simulink model "model_xs_gen_data"  (R2022a)
settings: Solver=ode45  StartTime=6.69  StopTime=11.57  FixedStep=0.056  MaxStep=0.001  RelTol=1e-3  AbsTol=1e-3  EnableMultiTasking=on
values from neighbouring files (symbols this model uses):
  Fout = [0 0 0 0 0 0 0 0 0.0168265476136 0.0188041 0.0188041 0.00691430249089 ... (1118 elements, 1118x1)]    [generated_data.mat]
  k = par(:, 2)    [ga_error.m]    (also in ga_error_gen_data.m; ga_optim.m = ParOpt(2); ga_optim_gen_data.m = ParOpt(2); ga_rv_optim.m = ParOpt(2))
  k1 = par(:, 3)    [ga_error.m]    (also in ga_error_gen_data.m; ga_optim.m = ParOpt(3); ga_optim_gen_data.m = ParOpt(3); ga_rv_optim.m = ParOpt(3))
  mu = par(:, 1)    [ga_error.m]    (also in ga_error_gen_data.m; ga_optim.m = ParOpt(1); ga_optim_gen_data.m = ParOpt(1); ga_rv_optim.m = ParOpt(1))
  S0 = Sd(1)    [Input_data.m]    (also in Input_data_sim.m; ga_optim.m; ga_optim_gen_data.m; ga_rv_optim.m)
  So = 100    [Input_data.m]    (also in Input_data_sim.m; ga_optim.m; ga_optim_gen_data.m; ga_rv_optim.m)
  tfe = tfeed    [ga_optim_gen_data.m]    (also in ga_rv_optim_gen_data.m)
  Vout = [1.35 1.35 1.35 1.35 1.35 1.35 1.35 1.35 1.35003365292 1.3500702132 1.35010340908 1.350112825 ... (1118 elements, 1118x1)]    [generated_data.mat]
  X0 = Xd(1)    [Input_data.m]    (also in Input_data_sim.m; ga_optim.m; ga_optim_gen_data.m; ga_rv_optim.m)
settings Model: ExtModeTrigMode=oneshot  ExtModeArmWhenConnect=off  Creator=Olympia  LastModifiedBy=Olympia
settings SolverCC: AutoScaleAbsTol=off  AlgebraicLoopSolver=TrustRegion
settings DataIOCC: SaveFormat=Array  SignalLoggingSaveFormat=ModelDataLogs  SaveOutput=off  SaveTime=off  ReturnWorkspaceOutputs=off
settings OptimizationCC: BlockReduction=off  BooleanDataType=off
settings DebuggingCC: SaveWithParameterizedLinksMsg=none  UnderspecifiedInitializationDetection=Classic  MergeDetectMultiDrivingBlocksExec=none  SignalResolutionControl=TryResolveAllWithWarning  MultiTaskDSMMsg=warning  MultiTaskCondExecSysMsg=none  UnconnectedInputMsg=warning  UnconnectedOutputMsg=warning  UnconnectedLineMsg=warning  SFMachineParentedDataDiag=warning  ArithmeticOperatorsInVariantConditions=warning
settings HardwareCC: TargetUnknown=on
settings ModelReferenceCC: PropagateSignalLabelsOutOfModel=off
settings SFSimCC: SimUseLocalCustomCode=off  CustomCodeUndefinedFunction=UseInterfaceOnly
settings RTWCC: RTWUseLocalCustomCode=off
settings CodeAppCC: StateflowObjectComments=on
settings GRTTargetCC: TargetLangStandard=C89/C90 (ANSI)  CombineOutputUpdateFcns=off  GRTInterface=on

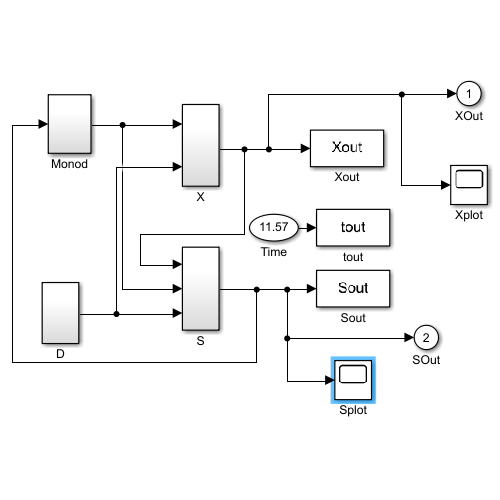
[thumbnail: Simulink's stored preview of the top-level diagram]
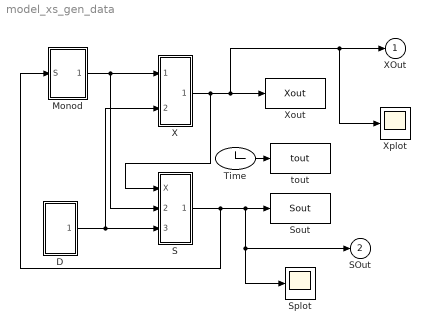
== system model_xs_gen_data ==
  D : Subsystem
  Monod : Subsystem
  S : Subsystem
  Sout : ToWorkspace  VariableName=Sout  SampleTime=-1
  Splot : Scope
  Time : Clock
  X : Subsystem
  Xout : ToWorkspace  VariableName=Xout  SampleTime=-1
  Xplot : Scope
  tout : ToWorkspace  VariableName=tout  SampleTime=-1
  XOut : Outport
  SOut : Outport  Port=2
  wires:
  X/1(XOut) -> Xout/1, Xplot/1, XOut/1, S/1(X)
  S/1(Sout) -> Monod/1(S), Sout/1, Splot/1, SOut/1
  Time/1 -> tout/1
  Monod/1(mu) -> X/1(mu), S/2(mu)
  D/1(out_1) -> S/3(F/V), X/2(F/V)

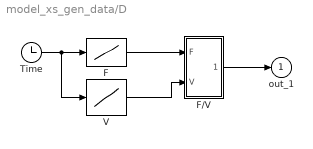
== system model_xs_gen_data/D ==
  F : Lookup  InputValues=tfe  Table=Fout
  F/V : Subsystem  mask(/){}
      mask help: Division of two scalars. y=u[1]/u[2]
      mask Help: Division of two scalars: y=u[1]/u[2]
      mask Display: disp('/')
  Time : Clock
  V : Lookup  InputValues=tfe  Table=Vout
  out_1 : Outport
  wires:
  F/V/1(out_1) -> out_1/1
  F/1 -> F/V/1(F)
  V/1 -> F/V/2(V)
  Time/1 -> F/1, V/1

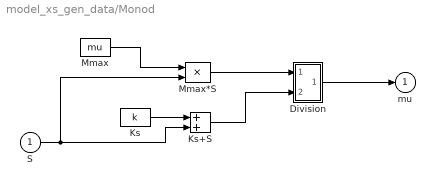
== system model_xs_gen_data/Monod ==
  S : Inport
  Division : Subsystem  mask(/){}
      mask help: Division of two scalars. y=u[1]/u[2]
      mask Help: Division of two scalars: y=u[1]/u[2]
      mask Display: disp('/')
  Ks : Constant  Value=k
  Ks+S : Sum  InputSameDT=on  SaturateOnIntegerOverflow=on  OutDataTypeStr=Inherit: Same as first input
  Mmax : Constant  Value=mu
  Mmax*S : Product  InputSameDT=on  RndMeth=Zero  SaturateOnIntegerOverflow=on  OutDataTypeStr=Inherit: Same as first input
  mu : Outport
  wires:
  Division/1(out_1) -> mu/1
  Mmax/1 -> Mmax*S/1
  Mmax*S/1 -> Division/1(Mmax*S)
  Ks+S/1 -> Division/2(Ks+S)
  Ks/1 -> Ks+S/1
  S/1 -> Ks+S/2, Mmax*S/2

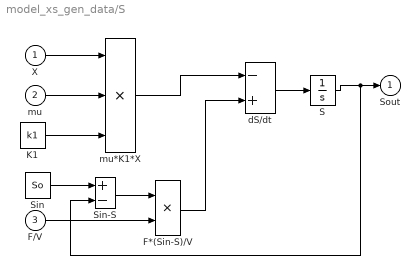
== system model_xs_gen_data/S ==
  X : Inport
  mu : Inport  Port=2
  F/V : Inport  Port=3
  F*(Sin-S)/V : Product  InputSameDT=on  RndMeth=Zero  SaturateOnIntegerOverflow=on  OutDataTypeStr=Inherit: Same as first input
  K1 : Constant  Value=k1
  S : Integrator  InitialCondition=S0  UpperSaturationLimit=1000  LowerSaturationLimit=0
  Sin : Constant  Value=So
  Sin-S : Sum  Inputs=+-  InputSameDT=on  SaturateOnIntegerOverflow=on  OutDataTypeStr=Inherit: Same as first input
  dS/dt : Sum  Inputs=-+  InputSameDT=on  SaturateOnIntegerOverflow=on  OutDataTypeStr=Inherit: Same as first input
  mu*K1*X : Product  Inputs=3  InputSameDT=on  RndMeth=Zero  SaturateOnIntegerOverflow=on  OutDataTypeStr=Inherit: Same as first input
  Sout : Outport
  wires:
  S/1 -> Sout/1, Sin-S/2
  Sin-S/1 -> F*(Sin-S)/V/1
  Sin/1 -> Sin-S/1
  X/1 -> mu*K1*X/1
  F/V/1 -> F*(Sin-S)/V/2
  mu*K1*X/1 -> dS/dt/1
  F*(Sin-S)/V/1 -> dS/dt/2
  dS/dt/1 -> S/1
  mu/1 -> mu*K1*X/2
  K1/1 -> mu*K1*X/3

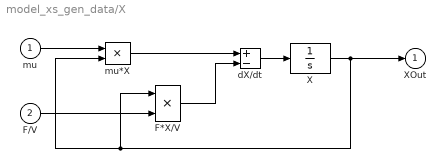
== system model_xs_gen_data/X ==
  mu : Inport
  F/V : Inport  Port=2
  F*X/V : Product  InputSameDT=on  RndMeth=Zero  SaturateOnIntegerOverflow=on  OutDataTypeStr=Inherit: Same as first input
  X : Integrator  InitialCondition=X0  UpperSaturationLimit=1000  LowerSaturationLimit=0
  dX/dt : Sum  Inputs=+-  InputSameDT=on  SaturateOnIntegerOverflow=on  OutDataTypeStr=Inherit: Same as first input
  mu*X : Product  InputSameDT=on  RndMeth=Zero  SaturateOnIntegerOverflow=on  OutDataTypeStr=Inherit: Same as first input
  XOut : Outport
  wires:
  F*X/V/1 -> dX/dt/2
  dX/dt/1 -> X/1
  mu*X/1 -> dX/dt/1
  mu/1 -> mu*X/1
  X/1 -> XOut/1, mu*X/2, F*X/V/1
  F/V/1 -> F*X/V/2

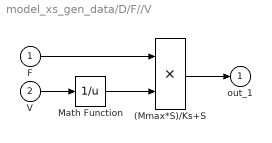
== system model_xs_gen_data/D/F//V ==
  F : Inport
  V : Inport  Port=2
  (Mmax*S)/Ks+S : Product  InputSameDT=on  RndMeth=Zero  SaturateOnIntegerOverflow=on  OutDataTypeStr=Inherit: Same as first input
  Math Function : Math  Operator=reciprocal  SignedPower=on
  out_1 : Outport
  wires:
  F/1 -> (Mmax*S)/Ks+S/1
  V/1 -> Math Function/1
  Math Function/1 -> (Mmax*S)/Ks+S/2
  (Mmax*S)/Ks+S/1 -> out_1/1

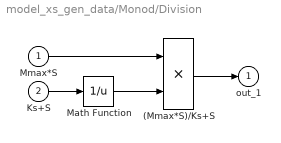
== system model_xs_gen_data/Monod/Division ==
  Mmax*S : Inport
  Ks+S : Inport  Port=2
  (Mmax*S)/Ks+S : Product  InputSameDT=on  RndMeth=Zero  SaturateOnIntegerOverflow=on  OutDataTypeStr=Inherit: Same as first input
  Math Function : Math  Operator=reciprocal  SignedPower=on
  out_1 : Outport
  wires:
  Mmax*S/1 -> (Mmax*S)/Ks+S/1
  Ks+S/1 -> Math Function/1
  Math Function/1 -> (Mmax*S)/Ks+S/2
  (Mmax*S)/Ks+S/1 -> out_1/1
